simulink model "sm_parts_custom_link"  (R2018b)
settings: Solver=VariableStepAuto  StartTime=0.0  StopTime=10.0  RelTol=1e-3  EnableMultiTasking=on
undefined symbols (not defined in the file): Local, X, Z
libraries: Multibody_Parts_Lib x7, sm_lib x2, nesl_utility x1
Description:
  | Copyright 2017-2018 The MathWorks, Inc.
settings Model: Creator=smiller  LastModifiedBy=smiller
settings DataIOCC: LimitDataPoints=on
settings OptimizationCC: LifeSpan=inf
settings DebuggingCC: AllowSymbolicDim=off  LibraryContextMissingDiagnostic=none  SFUnexpectedBacktrackingDiag=warning  SFNoUnconditionalDefaultTransitionDiag=warning  SFExecutionAtInitializationDiag=none
settings SFSimCC: SimUseLocalCustomCode=off
settings RTWCC: RTWUseLocalCustomCode=off
settings CodeAppCC: StateflowObjectComments=on
settings GRTTargetCC: TargetLangStandard=C89/C90 (ANSI)  GeneratePreprocessorConditionals=Disable all
settings ConfigComp: CovMetricSettings=dw  CovHtmlReporting=on  CovSaveCumulativeToWorkspaceVar=on  CovSaveSingleToWorkspaceVar=on  CovExternalEMLEnable=off  CovSFcnEnable=off
settings SimscapeCC: SimscapeNormalizeSystem=off  SimscapeLogType=all  SimscapeLogDataHistory=10000
settings ConfigurationSet: Description=SimMechanics 2G
settings ExplorerConfigSet: InternalSimMechanicsExplorerSettings="<ExplorerConfiguration><canonicalview>default</canonicalview><AnimationSetting><BasePlaybackSpeed>1.0</BasePlaybackSpeed><PlaybackSpeedFactor>1.0</PlaybackSpeedFactor></AnimationSetting><TilePanel><TileInfo><Tiles Columns=\"1\" Count=\"1\" Rows=\"1\"><Column Left=\"2\" Weight=\"1\"/><Column Left=\"563\"/><Row Top=\"2\" Weight=\"1\"/><Row Top=\"406\"/><Tile Height=\"1\" Width=\"1\" X=\"0\" Y=\"0\"/></Tiles></TileInfo><SceneInfo><SceneViewer><BGColor><R>1</R><G>1</G><B>1</B></BGColor><Camera><DoPerspective>off</DoPerspective><Position><X>-0.15311667332474177</X><Y>-0.86649769594677784</Y><Z>0.4741531998244457</Z></Position><Center><X>0.038361105534233914</X><Y>-0.0064592338598561394</Y><Z>0.0012154619197532468</Z></Center><Up><X>0.0084998133870717446</X><Y>0.48038242181850022</Y><Z>0.87701794849374537</Z></Up><ViewLimDist>1</ViewLimDist><YLim>0.039682415639306759</YLim><XLim>0.055454920083284377</XLim></Camera></SceneViewer></SceneInfo></TilePanel><MechEditorPanel><Cameras/><GfxPanelCameraMap/><VideoCreator><PlaybackSpeedRatio>1.0</PlaybackSpeedRatio><FrameRate>30</FrameRate><VideoFormat>Motion JPEG AVI</VideoFormat><FrameSize>auto</FrameSize></VideoCreator></MechEditorPanel></ExplorerConfiguration>"

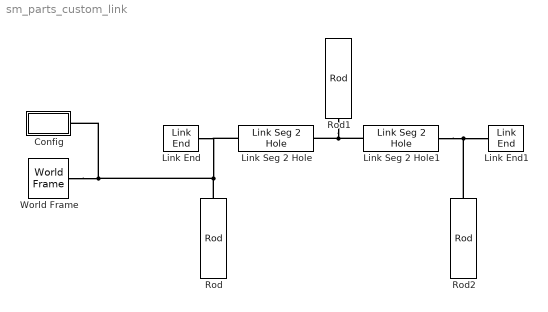
== system sm_parts_custom_link ==
  Config : Subsystem
  Link End : Multibody_Parts_Lib/Linkages/Link End  circ_radout=0.025/2  circ_radin=0.005  popup_holelr=-X  deg_1=90  deg_2=270  circ_len=0.01  circ_rho=7000  circ_color=[0.8 0.8 0.8]  circ_opc=1
      settings: SourceProductName=Simscape Multibody Parts Library
  Link End1 : Multibody_Parts_Lib/Linkages/Link End  circ_radout=0.025/2  circ_radin=0.005  popup_holelr=+X  deg_1=-90  deg_2=90  circ_len=0.01  circ_rho=7000  circ_color=[0 0.4 0.6]  circ_opc=1
      settings: SourceProductName=Simscape Multibody Parts Library
  Link Seg 2 Hole : Multibody_Parts_Lib/Linkages/Link Seg 2 Hole  link_len=0.05  link_width=0.025  link_radh=0.005  link_thickness=0.01  link_rho=7000  link_color=[0 0.4 0.6]  link_opc=1
      settings: SourceProductName=Simscape Multibody Parts Library
  Link Seg 2 Hole1 : Multibody_Parts_Lib/Linkages/Link Seg 2 Hole  link_len=0.03  link_width=0.025  link_radh=0.005  link_thickness=0.01  link_rho=7000  link_color=[0.8 0.8 0.8]  link_opc=1
      settings: SourceProductName=Simscape Multibody Parts Library
  Rod : Multibody_Parts_Lib/Basic/Rod  rod_rad=0.005  rod_len=0.025  rod_rho=7000  rod_color=[0.5 0.5 0.5]  rod_opc=1  popup_zori=Local +Z  popup_markings=None  mark_radius_range=[0.5 1.01]  mark_length_range=1.005  mark_angle_range=30  mark_color=[1 1 1]
      settings: SourceProductName=Simscape Multibody Parts Library
  Rod1 : Multibody_Parts_Lib/Basic/Rod  rod_rad=0.005  rod_len=0.025  rod_rho=7000  rod_color=[0.5 0.5 0.5]  rod_opc=1  popup_zori=Local +Z  popup_markings=None  mark_radius_range=[0.5 1.01]  mark_length_range=1.005  mark_angle_range=30  mark_color=[1 1 1]
      settings: SourceProductName=Simscape Multibody Parts Library
  Rod2 : Multibody_Parts_Lib/Basic/Rod  rod_rad=0.005  rod_len=0.025  rod_rho=7000  rod_color=[0.5 0.5 0.5]  rod_opc=1  popup_zori=Local +Z  popup_markings=None  mark_radius_range=[0.5 1.01]  mark_length_range=1.005  mark_angle_range=30  mark_color=[1 1 1]
      settings: SourceProductName=Simscape Multibody Parts Library
  World Frame : sm_lib/Frames and Transforms/World Frame
  connections:
  World Frame/RConn1 -- Link Seg 2 Hole/LConn1 -- Link End/LConn1 -- Rod/RConn1 -- Config/LConn1
  Link Seg 2 Hole1/LConn1 -- Link Seg 2 Hole/RConn1 -- Rod1/LConn1
  Link Seg 2 Hole1/RConn1 -- Rod2/RConn1 -- Link End1/LConn1

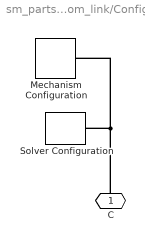
== system sm_parts_custom_link/Config ==
  Mechanism Configuration : sm_lib/Utilities/Mechanism Configuration  UniformGravity=Constant  GravityVector=[0 0 -9.80665]  GravityUnits=m/s^2  LinearizationDelta=0.001
  Solver Configuration : nesl_utility/Solver Configuration  PhysicalDomain=network_engine_domain  SubClassName=solver  LeftPortType=input  RightPortType=generic  Tones=[]  Harmonics=[]  SimulateNoise=off  Profile=off  UseLocalSampling=off  EnableSwitchedLinearOptims=on  FrequencyDomain=off  UseCCode=off  RelTol=0.001  AbsTol=1e-06  MinStep=1e-09  ToWorkspace=off  RevertToSquareIcSolve=off  NumHomotopyIterations=100  PhasorMode=off  PhasorModeNumHarmonics=1  DoDC=off  ResidualTolerance=1e-09  UseLocalSolver=off  LocalSolverChoice=NE_BACKWARD_EULER_ADVANCER  LocalSolverSampleTime=0.001  DoFixedCost=off  MaxNonlinIter=3  MaxModeIter=2  LinearAlgebra=Sparse  EquationFormulation=NE_TIME_EF  DelaysMemoryBudget=1024  AutomaticFiltering=on  FilteringTimeConstant=0.001  PartitionStorageMethod=AS_NEEDED  PartitionMemoryBudget=1024
  C : PMIOPort  Side=Left
  connections:
  Mechanism Configuration/RConn1 -- C/RConn1 -- Solver Configuration/RConn1
